simulink model "dofmodel"  (R2020b)
settings: Solver=VariableStepAuto  StartTime=0.0  StopTime=50  FixedStep=0.0001  RelTol=1e-3
values from neighbouring files (symbols this model uses):
  b = 1e-6    (= 1e-06)    [Variables.m]
  ct = 0.011586    [Variables.m]
  g = -9.81    [Variables.m]
  Jm = 0.000005    (= 5e-06)    [Variables.m]
  Ke = 1/3800    (= 0.000263157894737)    [Variables.m]
  Kt = Ke    (= 0.000263157894737)    [Variables.m]
  L = 0.0005    [Variables.m]
  m = 0.342    [Variables.m]
  Rm = 0.145    [Variables.m]
libraries: shared6dof x1, uavalgslib x1
settings Model: Creator=Josh_  LastModifiedBy=Josh_

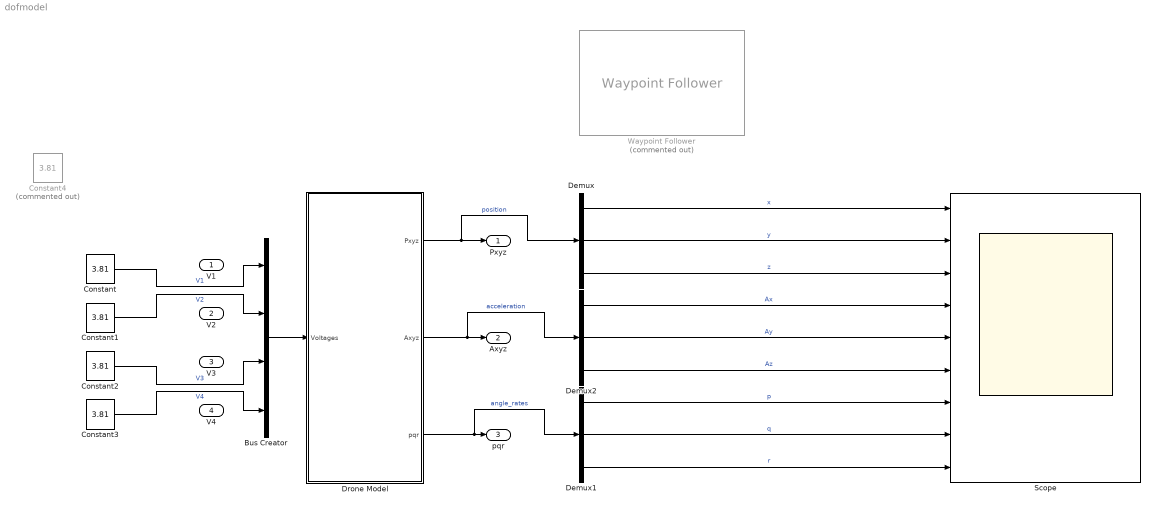
== system dofmodel ==
  V1 : Inport
  V2 : Inport  Port=2
  V3 : Inport  Port=3
  V4 : Inport  Port=4
  Bus Creator : BusCreator  Inputs=4
  Constant{,1..3} (4 alike) : Constant  Value=3.81
  Constant4 : Constant  Commented=on  Value=3.81
  Demux : Demux  Outputs=3
  Demux1 : Demux  Outputs=3
  Demux2 : Demux  Outputs=3
  Drone Model : Subsystem
  Scope : Scope  NumInputPorts=9
  Waypoint Follower : uavalgslib/Waypoint Follower  Commented=on  UAVType=multirotor  StartFrom=first  TransitionRadiusSource=internal  TransitionRadius=10  MinLookaheadDistance=0.1  YawInput=off  ShowCrossTrackErrorOutput=off  ShowStatusOutput=off  SimulateUsing=Interpreted execution
      settings: SourceProductBaseCode=UV
  Pxyz : Outport
  Axyz : Outport  Port=2
  pqr : Outport  Port=3
  wires:
  Demux/1 -> Scope/1  "x"
  Demux/2 -> Scope/2  "y"
  Demux/3 -> Scope/3  "z"
  Demux1/1 -> Scope/7  "p"
  Demux1/3 -> Scope/9  "r"
  Demux1/2 -> Scope/8  "q"
  Demux2/1 -> Scope/4  "Ax"
  Demux2/3 -> Scope/6  "Az"
  Demux2/2 -> Scope/5  "Ay"
  Drone Model/3(pqr) -> Demux1/1, pqr/1  "angle_rates"
  Drone Model/2(Axyz) -> Demux2/1, Axyz/1  "acceleration"
  Drone Model/1(Pxyz) -> Demux/1, Pxyz/1  "position"
  Bus Creator/1 -> Drone Model/1(Voltages)
  Constant3/1 -> Bus Creator/4  "V4"
  Constant2/1 -> Bus Creator/3  "V3"
  Constant1/1 -> Bus Creator/2  "V2"
  Constant/1 -> Bus Creator/1  "V1"

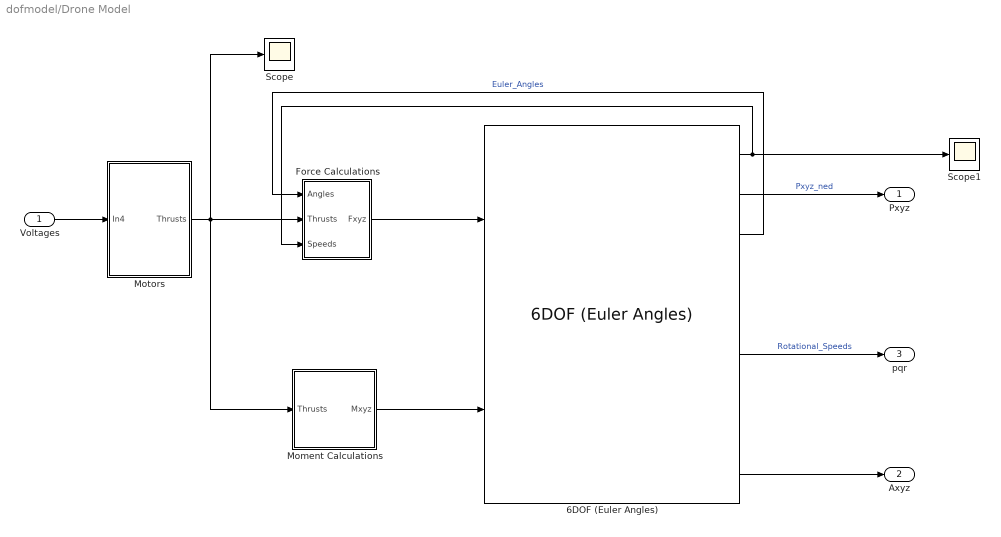
== system dofmodel/Drone Model ==
  Voltages : Inport
  6DOF (Euler Angles) : shared6dof/6DOF (Euler Angles)  units=Metric (MKS)  mtype=Fixed  rep=Euler Angles  xme_0=[0 0 0]  Vm_0=[0 0 0]  eul_0=[0 0 0]  pm_0=[0 0 0]  mass_0=m  mass_e=0.5  mass_f=2.0  inertia=eye(3)  inertia_e=eye(3)  inertia_f=2*eye(3)  k_quat=1.0  vre_flag=on  abi_flag=on  aMode=0  xme_statename=''  Vm_statename=''  eul_statename=''  quat_statename=''  pm_statename=''  mass_statename=''
      settings: SourceProductBaseCode=AE,PW,MT,UV,VE,VP
  Force Calculations : Subsystem
  Moment Calculations : Subsystem
  Motors : Subsystem
  Scope : Scope
  Scope1 : Scope
  Pxyz : Outport
  Axyz : Outport  Port=2
  pqr : Outport  Port=3
  wires:
  Moment Calculations/1(Mxyz) -> 6DOF (Euler Angles)/2
  Motors/1(Thrusts) -> Moment Calculations/1(Thrusts), Scope/1, Force Calculations/2(Thrusts)
  Voltages/1 -> Motors/1(In4)
  6DOF (Euler Angles)/2 -> Pxyz/1  "Pxyz_ned"
  6DOF (Euler Angles)/3 -> Force Calculations/1(Angles)  "Euler_Angles"
  Force Calculations/1(Fxyz) -> 6DOF (Euler Angles)/1
  6DOF (Euler Angles)/6 -> pqr/1  "Rotational_Speeds"
  6DOF (Euler Angles)/9 -> Axyz/1
  6DOF (Euler Angles)/1 -> Force Calculations/3(Speeds), Scope1/1

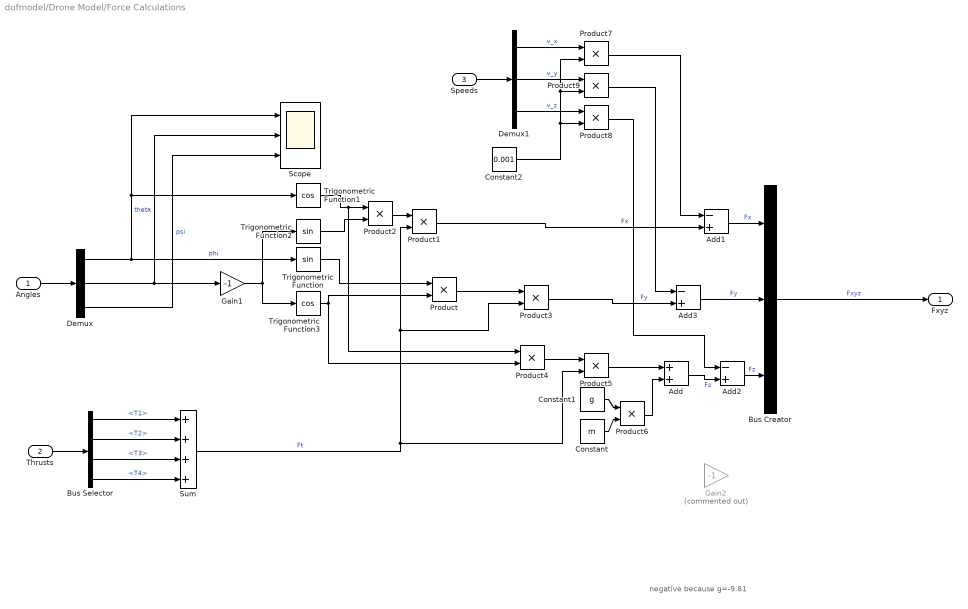
== system dofmodel/Drone Model/Force Calculations ==
  note: negative because g=-9.81
  Angles : Inport
  Thrusts : Inport  Port=2
  Speeds : Inport  Port=3
  Add : Sum
  Add1 : Sum  Inputs=-+
  Add2 : Sum  Inputs=-+
  Add3 : Sum  Inputs=-+
  Bus Creator : BusCreator  Inputs=3
  Bus Selector : BusSelector  OutputSignals=T1,T2,T3,T4
  Constant : Constant  Value=m
  Constant1 : Constant  Value=g
  Constant2 : Constant  Value=0.001
  Demux : Demux  Outputs=3
  Demux1 : Demux  Outputs=3
  Gain1 : Gain  Gain=-1
  Gain2 : Gain  Commented=on  Gain=-1
  Product{,1..9} (10 alike) : Product
  Scope : Scope  NumInputPorts=3
  Sum : Sum  Inputs=++++
  Trigonometric Function : Trigonometry
  Trigonometric Function1 : Trigonometry  Operator=cos
  Trigonometric Function2 : Trigonometry
  Trigonometric Function3 : Trigonometry  Operator=cos
  Fxyz : Outport
  wires:
  Constant/1 -> Product6/2
  Constant1/1 -> Product6/1
  Product5/1 -> Add/1
  Product4/1 -> Product5/1
  Product/1 -> Product3/1
  Demux/2 -> Gain1/1, Scope/2  "theta"
  Demux/1 -> Trigonometric Function/1, Trigonometric Function1/1, Scope/1  "phi"
  Angles/1 -> Demux/1
  Demux/3 -> Scope/3  "psi"
  Gain1/1 -> Trigonometric Function2/1, Trigonometric Function3/1
  Trigonometric Function1/1 -> Product4/1, Product2/1
  Trigonometric Function2/1 -> Product2/2
  Product2/1 -> Product1/1
  Sum/1 -> Product5/2, Product1/2, Product3/2  "Ft"
  Trigonometric Function/1 -> Product/1
  Trigonometric Function3/1 -> Product4/2, Product/2
  Thrusts/1 -> Bus Selector/1
  Bus Selector/1 -> Sum/1  "<T1>"
  Bus Selector/2 -> Sum/2  "<T2>"
  Bus Selector/3 -> Sum/3  "<T3>"
  Bus Selector/4 -> Sum/4  "<T4>"
  Bus Creator/1 -> Fxyz/1  "Fxyz"
  Product6/1 -> Add/2
  Speeds/1 -> Demux1/1
  Demux1/1 -> Product7/1  "v_x"
  Demux1/2 -> Product9/1  "v_y"
  Demux1/3 -> Product8/1  "v_z"
  Constant2/1 -> Product8/2, Product9/2, Product7/2
  Product1/1 -> Add1/2  "Fx"
  Add1/1 -> Bus Creator/1  "Fx"
  Add/1 -> Add2/2  "Fz"
  Add2/1 -> Bus Creator/3  "Fz"
  Add3/1 -> Bus Creator/2  "Fy"
  Product3/1 -> Add3/2  "Fy"
  Product8/1 -> Add2/1
  Product9/1 -> Add3/1
  Product7/1 -> Add1/1

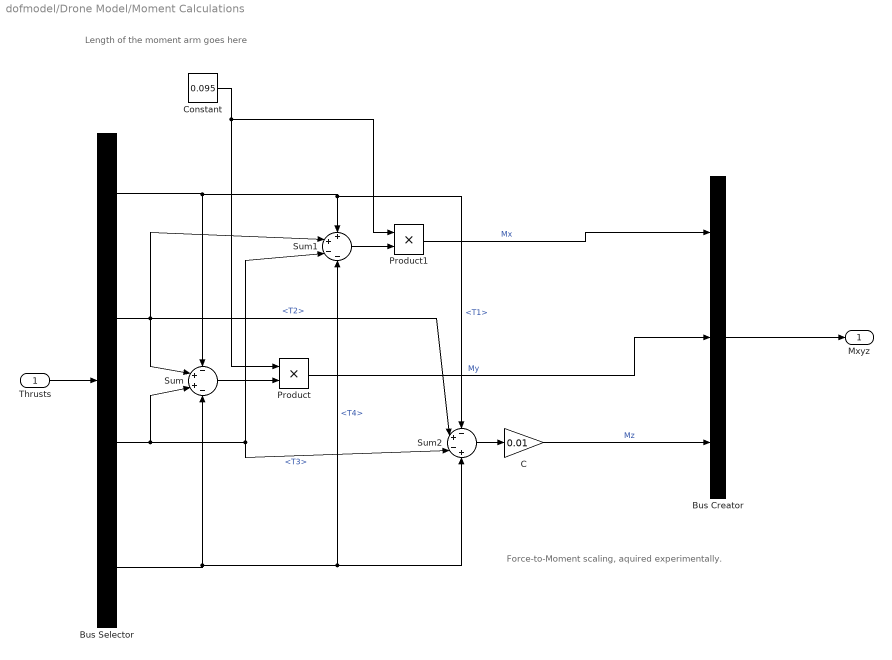
== system dofmodel/Drone Model/Moment Calculations ==
  note: Length of the moment arm goes here
  note: Force-to-Moment scaling, aquired experimentally.
  Thrusts : Inport
  Bus Creator : BusCreator  Inputs=3
  Bus Selector : BusSelector  OutputSignals=T1,T2,T3,T4
  C : Gain  Gain=0.01
  Constant : Constant  Value=0.095
  Product : Product
  Product1 : Product
  Sum : Sum  Inputs=-++-
  Sum1 : Sum  Inputs=++--
  Sum2 : Sum  Inputs=-+-+
  Mxyz : Outport
  wires:
  Bus Creator/1 -> Mxyz/1
  Bus Selector/1 -> Sum2/1, Sum1/1, Sum/1  "<T1>"
  Bus Selector/4 -> Sum2/4, Sum1/4, Sum/4  "<T4>"
  Thrusts/1 -> Bus Selector/1
  Bus Selector/2 -> Sum2/2, Sum/2, Sum1/2  "<T2>"
  Bus Selector/3 -> Sum1/3, Sum2/3, Sum/3  "<T3>"
  Sum2/1 -> C/1
  C/1 -> Bus Creator/3  "Mz"
  Sum/1 -> Product/2
  Constant/1 -> Product1/1, Product/1
  Sum1/1 -> Product1/2
  Product1/1 -> Bus Creator/1  "Mx"
  Product/1 -> Bus Creator/2  "My"

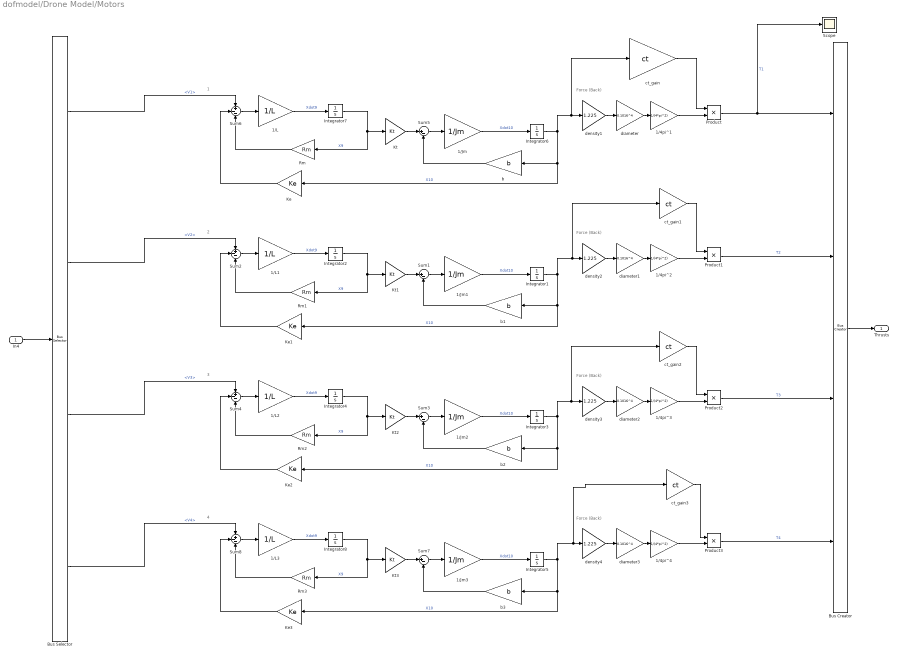
== system dofmodel/Drone Model/Motors ==
  note: Force (Back)
  note: 1
  note: 2
  note: Force (Back)
  note: 3
  note: Force (Back)
  note: 4
  note: Force (Back)
  In4 : Inport
  1/4pi^{1..4} (4 alike) : Gain  Gain=1/(4*pi^2)
  1/Jm{,1..3} (4 alike) : Gain  Gain=1/Jm
  1/L{,1..3} (4 alike) : Gain  Gain=1/L
  Bus Creator : BusCreator  Inputs=4
  Bus Selector : BusSelector  OutputSignals=V1,V2,V3,V4
  Integrator{1..8} (8 alike) : Integrator
  Ke{,1..3} (4 alike) : Gain  Gain=Ke
  Kt{,1..3} (4 alike) : Gain  Gain=Kt
  Product{,1..3} (4 alike) : Product
  Rm{,1..3} (4 alike) : Gain  Gain=Rm
  Scope : Scope
  Sum{1,3,5,7} (4 alike) : Sum  Inputs=|+-
  Sum{2,4,6,8} (4 alike) : Sum  Inputs=+--
  b{,1..3} (4 alike) : Gain  Gain=b
  ct_gain{,1..3} (4 alike) : Gain  Gain=ct
  density{1..4} (4 alike) : Gain  Gain=1.225
  diameter{,1..3} (4 alike) : Gain  Gain=0.1016^4
  Thrusts : Outport
  wires:
  In4/1 -> Bus Selector/1
  Sum5/1 -> 1/Jm/1
  Rm/1 -> Sum6/3
  1/Jm/1 -> Integrator6/1  "Xdot10"
  1/L/1 -> Integrator7/1  "Xdot9"
  diameter/1 -> 1/4pi^1/1
  Integrator6/1 -> density1/1, ct_gain/1, b/1, Ke/1  "X10"
  1/4pi^1/1 -> Product/2
  Integrator7/1 -> Rm/1, Kt/1  "X9"
  Kt/1 -> Sum5/1
  density1/1 -> diameter/1
  b/1 -> Sum5/2
  Sum6/1 -> 1/L/1
  Ke/1 -> Sum6/2
  Bus Creator/1 -> Thrusts/1
  b1/1 -> Sum1/2
  Ke1/1 -> Sum2/2
  Integrator2/1 -> Rm1/1, Kt1/1  "X9"
  density2/1 -> diameter1/1
  Sum2/1 -> 1/L1/1
  1/4pi^2/1 -> Product1/2
  1/Jm1/1 -> Integrator1/1  "Xdot10"
  diameter1/1 -> 1/4pi^2/1
  Kt1/1 -> Sum1/1
  1/L1/1 -> Integrator2/1  "Xdot9"
  Rm1/1 -> Sum2/3
  Sum1/1 -> 1/Jm1/1
  b2/1 -> Sum3/2
  Ke2/1 -> Sum4/2
  Integrator4/1 -> Rm2/1, Kt2/1  "X9"
  density3/1 -> diameter2/1
  Sum4/1 -> 1/L2/1
  1/4pi^3/1 -> Product2/2
  1/Jm2/1 -> Integrator3/1  "Xdot10"
  diameter2/1 -> 1/4pi^3/1
  Kt2/1 -> Sum3/1
  1/L2/1 -> Integrator4/1  "Xdot9"
  Rm2/1 -> Sum4/3
  Sum3/1 -> 1/Jm2/1
  b3/1 -> Sum7/2
  Ke3/1 -> Sum8/2
  Integrator8/1 -> Rm3/1, Kt3/1  "X9"
  density4/1 -> diameter3/1
  Sum8/1 -> 1/L3/1
  1/4pi^4/1 -> Product3/2
  1/Jm3/1 -> Integrator5/1  "Xdot10"
  diameter3/1 -> 1/4pi^4/1
  Kt3/1 -> Sum7/1
  1/L3/1 -> Integrator8/1  "Xdot9"
  Rm3/1 -> Sum8/3
  Sum7/1 -> 1/Jm3/1
  ct_gain/1 -> Product/1
  Product/1 -> Scope/1, Bus Creator/1  "T1"
  Product1/1 -> Bus Creator/2  "T2"
  Product2/1 -> Bus Creator/3  "T3"
  Product3/1 -> Bus Creator/4  "T4"
  Integrator1/1 -> ct_gain1/1, density2/1, b1/1, Ke1/1  "X10"
  ct_gain1/1 -> Product1/1
  Integrator3/1 -> ct_gain2/1, density3/1, b2/1, Ke2/1  "X10"
  ct_gain2/1 -> Product2/1
  Integrator5/1 -> ct_gain3/1, density4/1, b3/1, Ke3/1  "X10"
  ct_gain3/1 -> Product3/1
  Bus Selector/1 -> Sum6/1  "<V1>"
  Bus Selector/2 -> Sum2/1  "<V2>"
  Bus Selector/3 -> Sum4/1  "<V3>"
  Bus Selector/4 -> Sum8/1  "<V4>"
